simulink model "FLhighFidelityTiltingQuadrotor"  (R2022b)
settings: Solver=ode4  StartTime=0.0  StopTime=15  FixedStep=T_s  RelTol=1e-3
InitFcn:
  | run initFLhighFidelityTiltingQuadrotor
values from neighbouring files (symbols this model uses):
  kh1 = 1    [initFLhighFidelityTiltingQuadrotor.m]
  kh2 = 2    [initFLhighFidelityTiltingQuadrotor.m]
  Ts_st = settings.Ts_st    [initNMPChighFidelityTiltingQuadrotor.m]
  w_bar2_min = (0.01*prop.w_max).^2    [initFLhighFidelityTiltingQuadrotor.m]
  w_bar2_rest = tiltq.w_bar_hover_planar.^2    [initFLhighFidelityTiltingQuadrotor.m]
  w_bar_0 = w_bar_0(1:tiltq.N)    [highFidelityTiltingQuadrotorData.m]
undefined symbols (not defined in the file or in its folder): body, FL, prop, rad, s, tiltq
libraries: robotcorelib x4, simulink_extras x4, slpidlib x2, aerolibconvert2 x1, matrix_library x1
settings Model: PauseTimes=2  Creator=chen  LastModifiedBy=beniamino
settings SolverCC: AlgebraicLoopSolver=TrustRegion
settings DataIOCC: ReturnWorkspaceOutputs=off
settings DebuggingCC: UnconnectedInputMsg=warning  UnconnectedOutputMsg=warning  UnconnectedLineMsg=warning  SFMachineParentedDataDiag=warning  ArithmeticOperatorsInVariantConditions=warning
settings ModelReferenceCC: EnableRefExpFcnMdlSchedulingChecks=on
settings SFSimCC: SimUseLocalCustomCode=off  CustomCodeUndefinedFunction=UseInterfaceOnly
settings RTWCC: RTWUseLocalCustomCode=off  CheckMdlBeforeBuild=Error

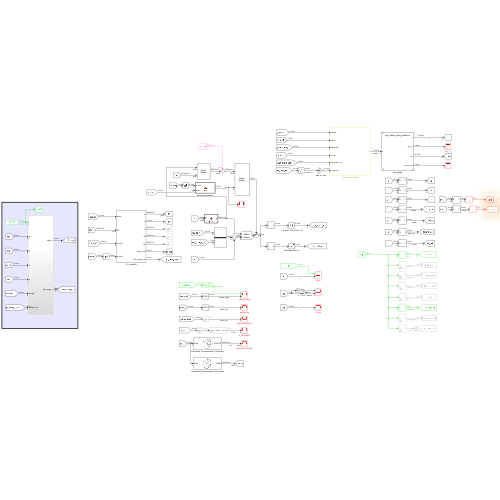
[thumbnail: Simulink's stored preview of the top-level diagram]
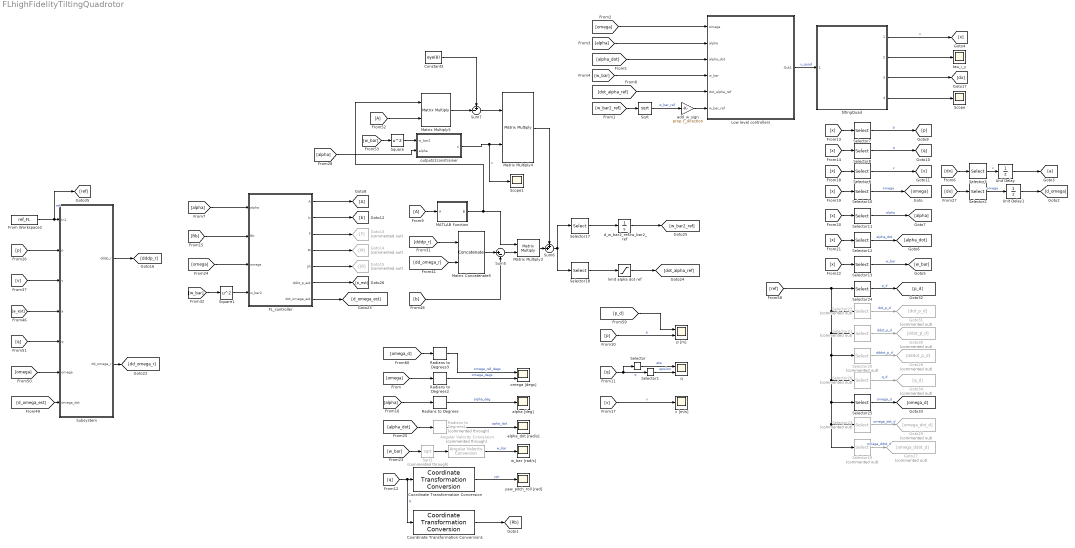
== system FLhighFidelityTiltingQuadrotor ==
  Angular Velocity Conversion : aerolibconvert2/Angular Velocity Conversion  Commented=through  IU=rad/s  OU=rpm
  Constant3 : Constant  Value=eye(8)
  Coordinate Transformation Conversion : robotcorelib/Coordinate Transformation Conversion  InputRepresentation=Quaternion  InputEulerSequence=ZYX  ShowTrVecInputPort=on  OutputRepresentation=Euler Angles  OutputEulerSequence=ZYX  ShowTrVecOutputPort=on  SimulateUsing=Code generation
  Coordinate Transformation Conversion1 : robotcorelib/Coordinate Transformation Conversion  InputRepresentation=Quaternion  InputEulerSequence=ZYX  ShowTrVecInputPort=on  OutputRepresentation=Rotation Matrix  OutputEulerSequence=ZYX  ShowTrVecOutputPort=on  SimulateUsing=Interpreted execution
  FL_controller : Subsystem
  From Workspace2 : FromWorkspace  VariableName=ref_FL  SampleTime=Ts_st
  From52 : From
  From9 : From
  Goto13 : Goto  Commented=on  GotoTag=F
  Goto14 : Goto  Commented=on  GotoTag=M
  Goto15 : Goto  Commented=on  GotoTag=JR
  Goto27 : Goto  Commented=on  GotoTag=omega_ddot_d
  Goto28 : Goto  Commented=on  GotoTag=dddot_p_d
  Goto29 : Goto  Commented=on  GotoTag=omega_dot_d
  Goto30 : Goto  Commented=on  GotoTag=ddot_p_d
  Goto31 : Goto  Commented=on  GotoTag=dot_p_d
  Goto34 : Goto  Commented=on  GotoTag=q_d
  Goto8 : Goto
  Low level controllers : Subsystem
  MATLAB Function : MATLAB Function  TreatAsAtomicUnit=on
  Matrix Concatenate5 : Concatenate  ConcatenateDimension=2
  Matrix Multiply3 : Product  Multiplication=Matrix(*)
  Matrix Multiply4 : Product  Multiplication=Matrix(*)
  Matrix Multiply5 : Product  Multiplication=Matrix(*)
  Radians to Degrees : simulink_extras/Transformations/Radians to Degrees
  Radians to Degrees1 : simulink_extras/Transformations/Radians to Degrees  Commented=through
  Radians to Degrees2 : simulink_extras/Transformations/Radians to Degrees
  Radians to Degrees3 : simulink_extras/Transformations/Radians to Degrees
  Scope : Scope
  Scope1 : Scope
  Selector : Selector  InputPortWidth=4  IndexOptions=Index vector (dialog)  Indices=1  OutputSizes=1
  Selector1 : Selector  InputPortWidth=4  IndexOptions=Index vector (dialog)  Indices=2:4  OutputSizes=1
  Selector10 : Selector  InputPortWidth=25  IndexOptions=Index vector (dialog)  Indices=11:13  OutputSizes=1
  Selector11 : Selector  InputPortWidth=25  IndexOptions=Index vector (dialog)  Indices=14:17  OutputSizes=1
  Selector12 : Selector  InputPortWidth=25  IndexOptions=Index vector (dialog)  Indices=18:21  OutputSizes=1
  Selector13 : Selector  InputPortWidth=25  IndexOptions=Index vector (dialog)  Indices=22:25  OutputSizes=1
  Selector17 : Selector  InputPortWidth=8  IndexOptions=Index vector (dialog)  Indices=1:4  OutputSizes=1
  Selector18 : Selector  InputPortWidth=8  IndexOptions=Index vector (dialog)  Indices=5:8  OutputSizes=1
  Selector19 : Selector  Commented=on  InputPortWidth=25  IndexOptions=Index vector (dialog)  Indices=23:25  OutputSizes=1
  Selector2 : Selector  InputPortWidth=25  IndexOptions=Index vector (dialog)  Indices=11:13  OutputSizes=1
  Selector20 : Selector  Commented=on  InputPortWidth=25  IndexOptions=Index vector (dialog)  Indices=20:22  OutputSizes=1
  Selector21 : Selector  Commented=on  InputPortWidth=25  IndexOptions=Index vector (dialog)  Indices=14:16  OutputSizes=1
  Selector22 : Selector  Commented=on  InputPortWidth=25  IndexOptions=Index vector (dialog)  Indices=8:10  OutputSizes=1
  Selector23 : Selector  Commented=on  InputPortWidth=25  IndexOptions=Index vector (dialog)  Indices=17:19  OutputSizes=1
  Selector24 : Selector  InputPortWidth=25  IndexOptions=Index vector (dialog)  Indices=1:3  OutputSizes=1
  Selector25 : Selector  InputPortWidth=25  IndexOptions=Index vector (dialog)  Indices=11:13  OutputSizes=1
  Selector26 : Selector  Commented=on  InputPortWidth=25  IndexOptions=Index vector (dialog)  Indices=4:7  OutputSizes=1
  Selector3 : Selector  InputPortWidth=25  IndexOptions=Index vector (dialog)  Indices=8:10  OutputSizes=1
  Selector7 : Selector  InputPortWidth=25  IndexOptions=Index vector (dialog)  Indices=1:3  OutputSizes=1
  Selector8 : Selector  InputPortWidth=25  IndexOptions=Index vector (dialog)  Indices=4:7  OutputSizes=1
  Selector9 : Selector  InputPortWidth=25  IndexOptions=Index vector (dialog)  Indices=8:10  OutputSizes=1
  Sqrt : Sqrt
  Sqrt1 : Sqrt  Commented=through
  Square : Math  Operator=square
  Square1 : Math  Operator=square
  Subsystem : Subsystem
  Sum5 : Sum  Inputs=|+-
  Sum6 : Sum  Inputs=++|
  Sum7 : Sum  Inputs=+-|
  Unit Delay : UnitDelay  SampleTime=-1  HasFrameUpgradeWarning=on
  Unit Delay1 : UnitDelay  SampleTime=-1  HasFrameUpgradeWarning=on
  add_w_sign : Gain  Gain=prop.c_direction
  alpha [deg] : Scope
  alpha_dot [rad/s] : Scope
  d_w_bar2_ref2w_bar2_ref : Integrator  InitialCondition=w_bar_0.^2  LimitOutput=on  UpperSaturationLimit=prop.w_max.^2  LowerSaturationLimit=prop.w_min.^2
  limit alpha dot ref : Saturate  UpperLimit=6  LowerLimit=-6
  omega [degs] : Scope  NumInputPorts=2
  outputs2constrainer : MATLAB Function  TreatAsAtomicUnit=on
  p [m] : Scope  NumInputPorts=2
  q : Scope  NumInputPorts=2
  tau_i_y : Scope
  tiltingQuad : Subsystem  ReferencedSubsystem=high_fidelity_tilting_quadrotor  p0=p_0  q0=q_0  v0=v_0  omega0=omega_0  alpha0=alpha_0  d_alpha_0=alpha_dot_0  bar_w0=w_bar_0  m_b=tiltq.m_b  beta=tiltq.beta  I_b=body.I  I_i=tiltq.I_i  c_direction=prop.c_direction  k_m=prop.k_m  k_t=prop.k_t  p_mot=tiltq.p_mot  min_alpha=tiltq.min_alpha  max_alpha=tiltq.max_alpha  min_d_alpha=tiltq.min_alpha_dot  max_d_alpha=tiltq.max_alpha_dot  min_bar_w=[prop.w_min prop.w_min -prop.w_max -prop.w_max]  max_bar_w=[prop.w_max prop.w_max -prop.w_min -prop.w_min]
  v [m/s] : Scope
  w_bar [rad/s] : Scope
  yaw_pitch_roll [rad] : Scope
  wires:
  tiltingQuad/3 -> [dx]
  tiltingQuad/1 -> [x]  "x"
  tiltingQuad/2 -> tau_i_y/1
  tiltingQuad/4 -> Scope/1
  [w_bar2_ref] -> Sqrt/1
  [omega] -> Low level controllers/1(omega)
  [alpha] -> Low level controllers/2(alpha)
  [alpha_dot] -> Low level controllers/3(alpha_dot)
  [w_bar] -> Low level controllers/4(w_bar)
  Sqrt/1 -> add_w_sign/1  "w_bar_ref"
  Low level controllers/1(Out1) -> tiltingQuad/1  "u_quad"
  [dot_alpha_ref] -> Low level controllers/5(dot_alpha_ref)
  Sum5/1 -> Matrix Multiply3/2
  Selector17/1 -> d_w_bar2_ref2w_bar2_ref/1
  MATLAB Function/1(B) -> Matrix Multiply5/1, Matrix Multiply3/1
  From Workspace2/1 -> [ref], Subsystem/1(In1)  "ref"
  [b] -> Sum5/2
  [p_d] -> p [m]/1
  [alpha] -> FL_controller/1(alpha)
  [q] -> Coordinate Transformation Conversion1/1, Coordinate Transformation Conversion/1  "q"
  Sqrt1/1 -> Angular Velocity Conversion/1
  [a_est] -> Subsystem/4(a)
  [p] -> Subsystem/2(p)
  Selector1/1 -> q/2  "epsilon"
  From9/1 -> MATLAB Function/1(A)
  Radians to Degrees2/1 -> omega [degs]/2  "omega_degs"
  Selector13/1 -> [w_bar]  "w_bar"
  Selector11/1 -> [alpha]  "alpha"
  [alpha] -> Radians to Degrees/1
  Subsystem/2(dd_omega_r) -> [dd_omega_r]
  Sum6/1 -> Selector18/1, Selector17/1
  [q] -> Selector1/1, Selector/1  "q"
  [w_bar] -> Square1/1
  [omega] -> Radians to Degrees2/1
  FL_controller/2(b) -> [b]
  [x] -> Selector10/1
  [x] -> Selector8/1
  Radians to Degrees/1 -> alpha [deg]/1  "alpha_deg"
  [v] -> Subsystem/3(v)
  Radians to Degrees1/1 -> alpha_dot [rad/s]/1  "apha_dot"
  Selector9/1 -> [v]  "v"
  [dd_omega_r] -> Matrix Concatenate5/2
  [x] -> Selector9/1
  Coordinate Transformation Conversion1/1 -> [Rb]
  FL_controller/1(A) -> Goto8/1
  FL_controller/3(F) -> Goto13/1
  Selector/1 -> q/1  "eta"
  Selector10/1 -> [omega]  "omega"
  Matrix Multiply5/1 -> Sum7/2
  Selector12/1 -> [alpha_dot]  "alpha_dot"
  Selector7/1 -> [p]  "p"
  [p] -> p [m]/2  "p"
  Matrix Concatenate5/1 -> Sum5/1
  [w_bar] -> Square/1
  Angular Velocity Conversion/1 -> w_bar [rad/s]/1  "w_bar"
  [x] -> Selector11/1
  Subsystem/1(dddp_r) -> [dddp_r]
  [x] -> Selector7/1
  Coordinate Transformation Conversion/1 -> yaw_pitch_roll [rad]/1  "ypr"
  Selector20/1 -> Goto28/1  "dddot_p_d"
  [Rb] -> FL_controller/2(Rb)
  From52/1 -> Matrix Multiply5/2
  [omega] -> FL_controller/3(omega)
  [x] -> Selector13/1
  Constant3/1 -> Sum7/1
  [alpha_dot] -> Radians to Degrees1/1
  Selector18/1 -> limit alpha dot ref/1
  FL_controller/5(JR) -> Goto15/1
  [d_omega_est] -> Subsystem/7(omega_dot)
  Selector24/1 -> [p_d]  "p_d"
  FL_controller/7(dot_omega_est) -> [d_omega_est]
  [x] -> Selector12/1
  [w_bar] -> Sqrt1/1
  [dddp_r] -> Matrix Concatenate5/1
  Matrix Multiply3/1 -> Sum6/2
  Sum7/1 -> Matrix Multiply4/1
  [v] -> v [m/s]/1  "v"
  Matrix Multiply4/1 -> Sum6/1
  [omega] -> Subsystem/6(omega)
  Selector26/1 -> Goto34/1  "q_d"
  outputs2constrainer/1(z) -> Scope1/1, Matrix Multiply4/2  "z"
  [ref] -> Selector21/1, Selector26/1, Selector25/1, Selector19/1, Selector23/1, Selector20/1, Selector22/1, Selector24/1
  Selector23/1 -> Goto29/1  "omega_dot_d"
  Selector8/1 -> [q]  "q"
  Selector21/1 -> Goto30/1  "ddot_p_d"
  FL_controller/6(ddot_p_est) -> [a_est]
  [q] -> Subsystem/5(q)
  FL_controller/4(M) -> Goto14/1
  Selector19/1 -> Goto27/1  "omega_ddot_d"
  [omega_d] -> Radians to Degrees3/1
  d_w_bar2_ref2w_bar2_ref/1 -> [w_bar2_ref]
  Selector25/1 -> [omega_d]  "omega_d"
  Selector22/1 -> Goto31/1  "dot_p_d"
  Radians to Degrees3/1 -> omega [degs]/1  "omega_ref_degs"
  add_w_sign/1 -> Low level controllers/6(w_bar_ref)
  Square/1 -> outputs2constrainer/1(w_bar2)
  Square1/1 -> FL_controller/4(w_bar2)
  limit alpha dot ref/1 -> [dot_alpha_ref]
  Selector2/1 -> Unit Delay1/1  "omega"
  [dx] -> Selector3/1
  Selector3/1 -> Unit Delay/1  "v"
  [dx] -> Selector2/1
  Unit Delay/1 -> [a]
  Unit Delay1/1 -> [d_omega]
  [alpha] -> outputs2constrainer/2(alpha)

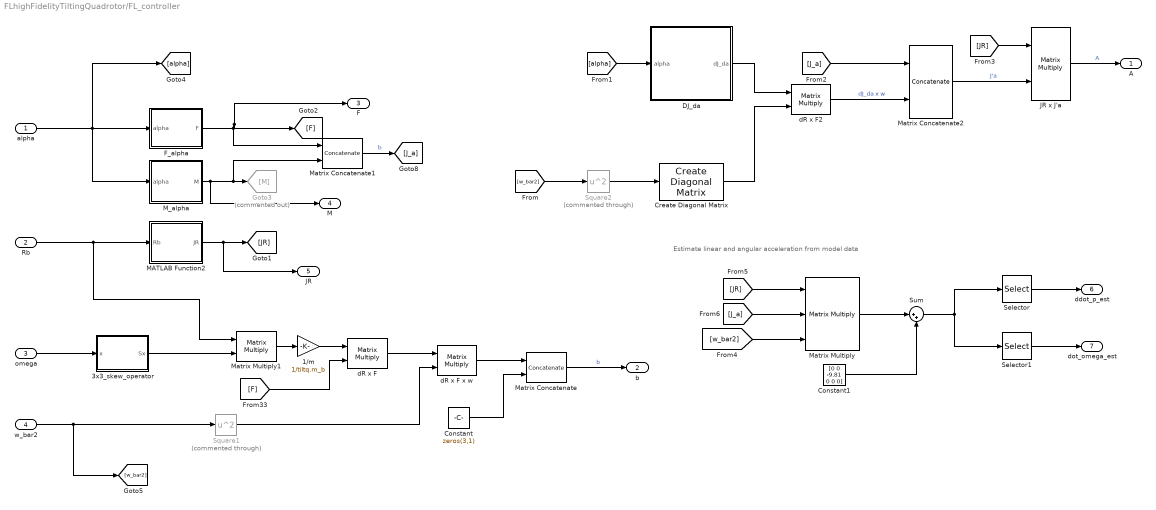
== system FLhighFidelityTiltingQuadrotor/FL_controller ==
  note: Estimate linear and angular acceleration from model data
  alpha : Inport
  Rb : Inport  Port=2
  omega : Inport  Port=3
  w_bar2 : Inport  Port=4
  1/m : Gain  Gain=1/tiltq.m_b
  3x3_skew_operator : MATLAB Function  TreatAsAtomicUnit=on
  Constant : Constant  Value=zeros(3,1)
  Constant1 : Constant  Value=[0 0 -9.81 0 0 0]
  Create Diagonal Matrix : matrix_library/Create Diagonal Matrix
      settings: LibrarySourceBlock=|
      | simulink/Matrix
      | Operations/Create Diagonal
      | Matrix
  DJ_da : MATLAB Function  TreatAsAtomicUnit=on  mask{c_t=prop.k_t, c_tau=prop.k_m, p_mot=tiltq.p_mot, beta=tiltq.beta, c_d=-prop.c_direction}
      mask prompts: c_t "thrust const"; c_tau "drag const"; p_mot "motor positions"; c_d "spinning directions"
  F_alpha : MATLAB Function  TreatAsAtomicUnit=on  mask{beta=tiltq.beta, c_t=prop.k_t}
      mask prompts: c_t "thrust_coeff"
  Goto3 : Goto  Commented=on  GotoTag=M
  JR x J'a : Product  Multiplication=Matrix(*)
  MATLAB Function2 : MATLAB Function  TreatAsAtomicUnit=on  mask{m=tiltq.m_b, Ib=body.I}
      mask prompts: m "mass"; Ib "Body inertia"
  M_alpha : MATLAB Function  TreatAsAtomicUnit=on  mask{beta=tiltq.beta, theta=tiltq.theta, c_t=prop.k_t, c_tau=prop.k_m, c_direction=-prop.c_direction, p_mot=tiltq.p_mot}
      mask prompts: c_t "thrust coeff"; c_tau "drag coeff"; c_direction "spinning dir"; p_mot "motor pos"
  Matrix Concatenate : Concatenate  Mode=Multidimensional array
  Matrix Concatenate1 : Concatenate  Mode=Multidimensional array
  Matrix Concatenate2 : Concatenate  Mode=Multidimensional array  ConcatenateDimension=2
  Matrix Multiply : Product  Inputs=3  Multiplication=Matrix(*)
  Matrix Multiply1 : Product  Multiplication=Matrix(*)
  Selector : Selector  InputPortWidth=6  IndexOptions=Index vector (dialog)  Indices=1:3  OutputSizes=1
  Selector1 : Selector  InputPortWidth=6  IndexOptions=Index vector (dialog)  Indices=4:6  OutputSizes=1
  Square1 : Math  Commented=through  Operator=square
  Square2 : Math  Commented=through  Operator=square
  Sum : Sum  Inputs=|++
  dR x F : Product  Multiplication=Matrix(*)
  dR x F x w : Product  Multiplication=Matrix(*)
  dR x F2 : Product  Multiplication=Matrix(*)
  A : Outport  PortDimensions=[6 8]
  b : Outport  Port=2  PortDimensions=6
  F : Outport  Port=3
  M : Outport  Port=4
  JR : Outport  Port=5
  ddot_p_est : Outport  Port=6
  dot_omega_est : Outport  Port=7
  wires:
  dR x F/1 -> dR x F x w/1
  dR x F x w/1 -> Matrix Concatenate/1
  Constant/1 -> Matrix Concatenate/2
  1/m/1 -> dR x F/1
  Rb/1 -> Matrix Multiply1/1, MATLAB Function2/1(Rb)
  M_alpha/1(M) -> M/1, Matrix Concatenate1/2, Goto3/1
  3x3_skew_operator/1(Sx) -> Matrix Multiply1/2
  alpha/1 -> [alpha], M_alpha/1(alpha), F_alpha/1(alpha)
  omega/1 -> 3x3_skew_operator/1(x)
  Square1/1 -> dR x F x w/2
  Matrix Concatenate1/1 -> [J_a]  "b"
  [F] -> dR x F/2
  w_bar2/1 -> [w_bar2], Square1/1
  MATLAB Function2/1(JR) -> JR/1, [JR]
  F_alpha/1(F) -> F/1, [F], Matrix Concatenate1/1
  Matrix Multiply1/1 -> 1/m/1
  Matrix Concatenate/1 -> b/1  "b"
  [J_a] -> Matrix Concatenate2/1
  Matrix Concatenate2/1 -> JR x J'a/2  "J'a"
  [JR] -> JR x J'a/1
  JR x J'a/1 -> A/1  "A"
  [w_bar2] -> Square2/1
  DJ_da/1(dJ_da) -> dR x F2/1
  [alpha] -> DJ_da/1(alpha)
  dR x F2/1 -> Matrix Concatenate2/2  "dJ_da x w"
  Square2/1 -> Create Diagonal Matrix/1
  Create Diagonal Matrix/1 -> dR x F2/2
  [w_bar2] -> Matrix Multiply/3
  [JR] -> Matrix Multiply/1
  [J_a] -> Matrix Multiply/2
  Matrix Multiply/1 -> Sum/1
  Selector/1 -> ddot_p_est/1
  Selector1/1 -> dot_omega_est/1
  Sum/1 -> Selector/1, Selector1/1
  Constant1/1 -> Sum/2

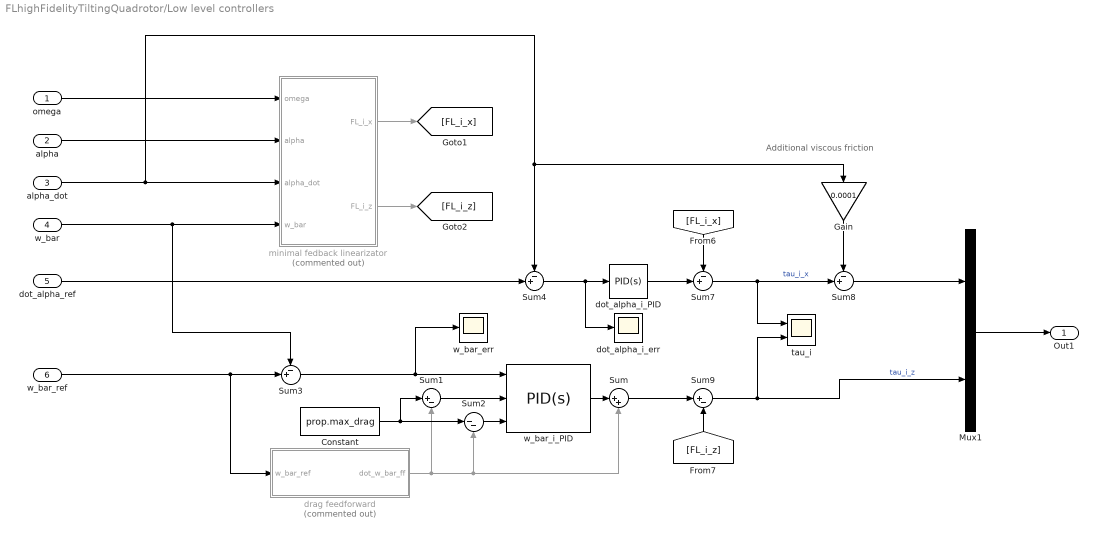
== system FLhighFidelityTiltingQuadrotor/Low level controllers ==
  note: Additional viscous friction
  omega : Inport
  alpha : Inport  Port=2
  alpha_dot : Inport  Port=3
  w_bar : Inport  Port=4
  dot_alpha_ref : Inport  Port=5
  w_bar_ref : Inport  Port=6
  Constant : Constant  Value=prop.max_drag
  Gain : Gain  Gain=0.0001
  Mux1 : Mux  Inputs=2
  Sum : Sum  Inputs=|++
  Sum1 : Sum  Inputs=|+-
  Sum2 : Sum  Inputs=|--
  Sum{3..4,7..8} (4 alike) : Sum  Inputs=-+|
  Sum9 : Sum  Inputs=|+-
  dot_alpha_i_PID : slpidlib/PID Controller  Controller=PID  Form=Parallel  TimeDomain=Continuous-time  UseExternalTs=off  SampleTime=-1  IntegratorMethod=Forward Euler  FilterMethod=Forward Euler  ControllerParametersSource=internal  P=0.01  I=0.1  UseKiTs=off  D=0.00001  N=100  UseFilter=on  TunerSelectOption=Transfer Function Based (PID Tuner App)  InitialConditionSource=internal  InitialConditionForIntegrator=0  InitialConditionForFilter=0  DifferentiatorICPrevScaledInput=0  ExternalReset=none  TrackingMode=off  Kt=1  LimitOutput=off  SatLimitsSource=internal  UpperSaturationLimit=6  LowerSaturationLimit=-6  LinearizeAsGain=on  AntiWindupMode=back-calculation  Kb=1  LimitIntegrator=off  UpperIntegratorSaturationLimit=inf  LowerIntegratorSaturationLimit=-inf  POutMin=[]  POutMax=[]  IOutMin=[]  IOutMax=[]  DOutMin=[]  DOutMax=[]  NOutMin=[]  NOutMax=[]  SumOutMin=[]  SumOutMax=[]  SaturationOutMin=[]  SaturationOutMax=[]  PParamMin=[]  PParamMax=[]  IParamMin=[]  IParamMax=[]  DParamMin=[]  DParamMax=[]  NParamMin=[]  NParamMax=[]  KbParamMin=[]  KbParamMax=[]  KtParamMin=[]  KtParamMax=[]  KbOutMin=[]  KbOutMax=[]  KtOutMin=[]  KtOutMax=[]  IntegratorOutMin=[]  IntegratorOutMax=[]  FilterOutMin=[]  FilterOutMax=[]  SumI1OutMin=[]  SumI1OutMax=[]  SumI2OutMin=[]  SumI2OutMax=[]  SumI3OutMin=[]  SumI3OutMax=[]  SumI4OutMin=[]  SumI4OutMax=[]  SumDOutMin=[]  SumDOutMax=[]  DifferentiatorOutMin=[]  DifferentiatorOutMax=[]  FilterDiffOutCoefMin=[]  FilterDiffOutCoefMax=[]  ReciprocalOutMin=[]  ReciprocalOutMax=[]  SumDenOutMin=[]  SumDenOutMax=[]  SumNumOutMin=[]  SumNumOutMax=[]  DivideOutMin=[]  DivideOutMax=[]  UdiffTsProdOutMin=[]  UdiffTsProdOutMax=[]  NTsProdOutMin=[]  NTsProdOutMax=[]  UintegralTsProdOutMin=[]  UintegralTsProdOutMax=[]  UngainTsProdOutMin=[]  UngainTsProdOutMax=[]  ClampingZeroOutDataTypeStr=Inherit: Inherit via back propagation  ClampingZeroOutMin=[]  ClampingZeroOutMax=[]  FilterDenConstantOutDataTypeStr=Inherit: Inherit via back propagation  FilterDenConstantOutMin=[]  FilterDenConstantOutMax=[]  PCopyOutDataTypeStr=Inherit: Inherit via back propagation  PCopyOutMin=[]  PCopyOutMax=[]  NCopyOutDataTypeStr=Inherit: Inherit via back propagation  NCopyOutMin=[]  NCopyOutMax=[]  IntegratorContinuousStateAttributes=''  IntegratorStateMustResolveToSignalObject=off  IntegratorRTWStateStorageClass=Auto  FilterContinuousStateAttributes=''  FilterStateMustResolveToSignalObject=off  FilterRTWStateStorageClass=Auto  ParallelPVariant=InternalParameters  IdealPVariant=Disabled  IVariant=InternalParameters  DVariant=InternalParameters  IntegratorVariant=Continuous  SatVariant=Disabled  AWVariant=Passthrough  PCopyVariant=Disabled  TRVariant=Disabled  FdbkBlocksVariant=Forward  IdealPFdbkVariant=Disabled  SatFdbkVariant=Disabled  DerivativeFilterVariant=ContFilter  NVariant=InternalParameters  NCopyVariant=Disabled  FilterICVariant=InternalICsFilter  IntegratorICVariant=InternalICs  ExternalResetVariant=Disabled  TRSumVariant=Passthrough  SumFdbkVariant=Disabled  SumVariant=Sum_PID  TsampFilterVariant=InternalTs  TsampNgainVariant=Passthrough  TsampIntegralVariant=Passthrough  ExternalSaturationOutDataTypeStr=Inherit: Same as second input
  dot_alpha_i_err : Scope
  drag feedforward : MATLAB Function  Commented=on  TreatAsAtomicUnit=on  mask{k_m=prop.k_m}
      mask prompts: k_m "motor drag constant"
  minimal fedback linearizator : MATLAB Function  Commented=on  TreatAsAtomicUnit=on  mask{N=tiltq.N, I_i=tiltq.I_i, beta=tiltq.beta}
      mask prompts: N "number of propellers"; I_i "propeller + rotor inertia matrix"; beta "propeller tilting planes angles"
  tau_i : Scope  NumInputPorts=2
  w_bar_err : Scope
  w_bar_i_PID : slpidlib/PID Controller  Controller=PID  Form=Parallel  TimeDomain=Continuous-time  UseExternalTs=off  SampleTime=-1  IntegratorMethod=Forward Euler  FilterMethod=Forward Euler  ControllerParametersSource=internal  P=0.01  I=0.1  UseKiTs=on  D=0.00001  N=100  UseFilter=on  TunerSelectOption=Transfer Function Based (PID Tuner App)  InitialConditionSource=internal  InitialConditionForIntegrator=0  InitialConditionForFilter=0  DifferentiatorICPrevScaledInput=0  ExternalReset=none  TrackingMode=off  Kt=1  LimitOutput=on  SatLimitsSource=external  UpperSaturationLimit=inf  LowerSaturationLimit=-inf  LinearizeAsGain=on  AntiWindupMode=back-calculation  Kb=10  LimitIntegrator=off  UpperIntegratorSaturationLimit=inf  LowerIntegratorSaturationLimit=-inf  POutMin=[]  POutMax=[]  IOutMin=[]  IOutMax=[]  DOutMin=[]  DOutMax=[]  NOutMin=[]  NOutMax=[]  SumOutMin=[]  SumOutMax=[]  SaturationOutMin=[]  SaturationOutMax=[]  PParamMin=[]  PParamMax=[]  IParamMin=[]  IParamMax=[]  DParamMin=[]  DParamMax=[]  NParamMin=[]  NParamMax=[]  KbParamMin=[]  KbParamMax=[]  KtParamMin=[]  KtParamMax=[]  KbOutMin=[]  KbOutMax=[]  KtOutMin=[]  KtOutMax=[]  IntegratorOutMin=[]  IntegratorOutMax=[]  FilterOutMin=[]  FilterOutMax=[]  SumI1OutMin=[]  SumI1OutMax=[]  SumI2OutMin=[]  SumI2OutMax=[]  SumI3OutMin=[]  SumI3OutMax=[]  SumI4OutMin=[]  SumI4OutMax=[]  SumDOutMin=[]  SumDOutMax=[]  DifferentiatorOutMin=[]  DifferentiatorOutMax=[]  FilterDiffOutCoefMin=[]  FilterDiffOutCoefMax=[]  ReciprocalOutMin=[]  ReciprocalOutMax=[]  SumDenOutMin=[]  SumDenOutMax=[]  SumNumOutMin=[]  SumNumOutMax=[]  DivideOutMin=[]  DivideOutMax=[]  UdiffTsProdOutMin=[]  UdiffTsProdOutMax=[]  NTsProdOutMin=[]  NTsProdOutMax=[]  UintegralTsProdOutMin=[]  UintegralTsProdOutMax=[]  UngainTsProdOutMin=[]  UngainTsProdOutMax=[]  ClampingZeroOutDataTypeStr=Inherit: Inherit via back propagation  ClampingZeroOutMin=[]  ClampingZeroOutMax=[]  FilterDenConstantOutDataTypeStr=Inherit: Inherit via back propagation  FilterDenConstantOutMin=[]  FilterDenConstantOutMax=[]  PCopyOutDataTypeStr=Inherit: Inherit via back propagation  PCopyOutMin=[]  PCopyOutMax=[]  NCopyOutDataTypeStr=Inherit: Inherit via back propagation  NCopyOutMin=[]  NCopyOutMax=[]  IntegratorContinuousStateAttributes=''  IntegratorStateMustResolveToSignalObject=off  IntegratorRTWStateStorageClass=Auto  FilterContinuousStateAttributes=''  FilterStateMustResolveToSignalObject=off  FilterRTWStateStorageClass=Auto  ParallelPVariant=InternalParameters  IdealPVariant=Disabled  IVariant=InternalParameters  DVariant=InternalParameters  IntegratorVariant=Continuous  SatVariant=External  AWVariant=BackCalculation  PCopyVariant=Disabled  TRVariant=Disabled  FdbkBlocksVariant=Forward  IdealPFdbkVariant=Disabled  SatFdbkVariant=Disabled  DerivativeFilterVariant=ContFilter  NVariant=InternalParameters  NCopyVariant=Disabled  FilterICVariant=InternalICsFilter  IntegratorICVariant=InternalICs  ExternalResetVariant=Disabled  TRSumVariant=Passthrough  SumFdbkVariant=Disabled  SumVariant=Sum_PID  TsampFilterVariant=InternalTs  TsampNgainVariant=Passthrough  TsampIntegralVariant=Passthrough  ExternalSaturationOutDataTypeStr=Inherit: Same as second input
  Out1 : Outport
  wires:
  Sum2/1 -> w_bar_i_PID/3
  w_bar_i_PID/1 -> Sum/1
  minimal fedback linearizator/1(FL_i_x) -> [FL_i_x]
  Sum8/1 -> Mux1/1
  dot_alpha_i_PID/1 -> Sum7/2
  alpha_dot/1 -> Gain/1, Sum4/1, minimal fedback linearizator/3(alpha_dot)
  Sum4/1 -> dot_alpha_i_err/1, dot_alpha_i_PID/1
  [FL_i_z] -> Sum9/2
  minimal fedback linearizator/2(FL_i_z) -> [FL_i_z]
  alpha/1 -> minimal fedback linearizator/2(alpha)
  Sum9/1 -> tau_i/2, Mux1/2  "tau_i_z"
  omega/1 -> minimal fedback linearizator/1(omega)
  Sum/1 -> Sum9/1
  Sum1/1 -> w_bar_i_PID/2
  [FL_i_x] -> Sum7/1
  Mux1/1 -> Out1/1
  Sum3/1 -> w_bar_err/1, w_bar_i_PID/1
  w_bar/1 -> Sum3/1, minimal fedback linearizator/4(w_bar)
  dot_alpha_ref/1 -> Sum4/2
  Sum7/1 -> tau_i/1, Sum8/2  "tau_i_x"
  Gain/1 -> Sum8/1
  w_bar_ref/1 -> Sum3/2, drag feedforward/1(w_bar_ref)
  drag feedforward/1(dot_w_bar_ff) -> Sum/2, Sum2/2, Sum1/2
  Constant/1 -> Sum2/1, Sum1/1

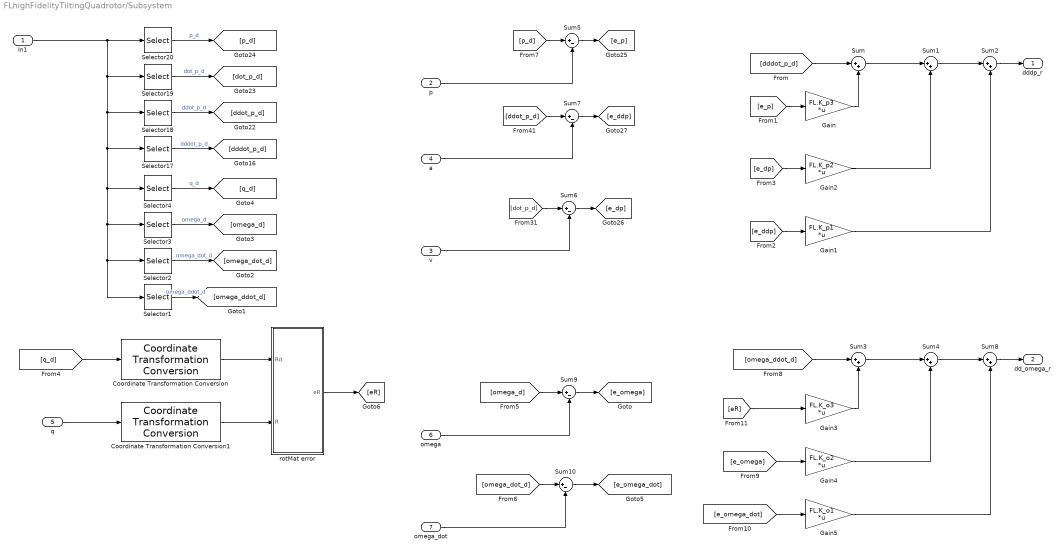
== system FLhighFidelityTiltingQuadrotor/Subsystem ==
  In1 : Inport
  p : Inport  Port=2
  v : Inport  Port=3
  a : Inport  Port=4
  q : Inport  Port=5
  omega : Inport  Port=6
  omega_dot : Inport  Port=7
  Coordinate Transformation Conversion : robotcorelib/Coordinate Transformation Conversion  InputRepresentation=Quaternion  InputEulerSequence=ZYX  ShowTrVecInputPort=on  OutputRepresentation=Rotation Matrix  OutputEulerSequence=ZYX  ShowTrVecOutputPort=on  SimulateUsing=Interpreted execution
  Coordinate Transformation Conversion1 : robotcorelib/Coordinate Transformation Conversion  InputRepresentation=Quaternion  InputEulerSequence=ZYX  ShowTrVecInputPort=on  OutputRepresentation=Rotation Matrix  OutputEulerSequence=ZYX  ShowTrVecOutputPort=on  SimulateUsing=Interpreted execution
  Gain : Gain  Gain=FL.K_p3  Multiplication=Matrix(K*u) (u vector)
  Gain1 : Gain  Gain=FL.K_p1  Multiplication=Matrix(K*u) (u vector)
  Gain2 : Gain  Gain=FL.K_p2  Multiplication=Matrix(K*u) (u vector)
  Gain3 : Gain  Gain=FL.K_o3  Multiplication=Matrix(K*u) (u vector)
  Gain4 : Gain  Gain=FL.K_o2  Multiplication=Matrix(K*u) (u vector)
  Gain5 : Gain  Gain=FL.K_o1  Multiplication=Matrix(K*u) (u vector)
  Selector1 : Selector  InputPortWidth=25  IndexOptions=Index vector (dialog)  Indices=23:25  OutputSizes=1
  Selector17 : Selector  InputPortWidth=25  IndexOptions=Index vector (dialog)  Indices=20:22  OutputSizes=1
  Selector18 : Selector  InputPortWidth=25  IndexOptions=Index vector (dialog)  Indices=14:16  OutputSizes=1
  Selector19 : Selector  InputPortWidth=25  IndexOptions=Index vector (dialog)  Indices=8:10  OutputSizes=1
  Selector2 : Selector  InputPortWidth=25  IndexOptions=Index vector (dialog)  Indices=17:19  OutputSizes=1
  Selector20 : Selector  InputPortWidth=25  IndexOptions=Index vector (dialog)  Indices=1:3  OutputSizes=1
  Selector3 : Selector  InputPortWidth=25  IndexOptions=Index vector (dialog)  Indices=11:13  OutputSizes=1
  Selector4 : Selector  InputPortWidth=25  IndexOptions=Index vector (dialog)  Indices=4:7  OutputSizes=1
  Sum{,1..4,8} (6 alike) : Sum  Inputs=|++
  Sum{5..7,9..10} (5 alike) : Sum  Inputs=|+-
  rotMat error : MATLAB Function  TreatAsAtomicUnit=on
  dddp_r : Outport
  dd_omega_r : Outport  Port=2
  wires:
  Selector19/1 -> [dot_p_d]  "dot_p_d"
  a/1 -> Sum7/2
  [p_d] -> Sum5/1
  p/1 -> Sum5/2
  [ddot_p_d] -> Sum7/1
  Selector18/1 -> [ddot_p_d]  "ddot_p_d"
  Sum6/1 -> [e_dp]
  [dot_p_d] -> Sum6/1
  v/1 -> Sum6/2
  Sum7/1 -> [e_ddp]
  Sum5/1 -> [e_p]
  Selector17/1 -> [dddot_p_d]  "dddot_p_d"
  Selector20/1 -> [p_d]  "p_d"
  [dddot_p_d] -> Sum/1
  [e_p] -> Gain/1
  Gain/1 -> Sum/2
  Sum/1 -> Sum1/1
  [e_ddp] -> Gain1/1
  Gain1/1 -> Sum2/2
  [e_dp] -> Gain2/1
  Sum1/1 -> Sum2/1
  Gain2/1 -> Sum1/2
  Sum2/1 -> dddp_r/1
  Sum8/1 -> dd_omega_r/1
  Gain3/1 -> Sum3/2
  Gain5/1 -> Sum8/2
  Sum3/1 -> Sum4/1
  Gain4/1 -> Sum4/2
  Sum4/1 -> Sum8/1
  [omega_ddot_d] -> Sum3/1
  Selector4/1 -> [q_d]  "q_d"
  Selector1/1 -> [omega_ddot_d]  "omega_ddot_d"
  Selector2/1 -> [omega_dot_d]  "omega_dot_d"
  In1/1 -> Selector18/1, Selector4/1, Selector3/1, Selector1/1, Selector2/1, Selector17/1, Selector19/1, Selector20/1
  Selector3/1 -> [omega_d]  "omega_d"
  [omega_d] -> Sum9/1
  omega/1 -> Sum9/2
  [omega_dot_d] -> Sum10/1
  omega_dot/1 -> Sum10/2
  Sum9/1 -> [e_omega]
  Sum10/1 -> [e_omega_dot]
  [e_omega] -> Gain4/1
  [e_omega_dot] -> Gain5/1
  [q_d] -> Coordinate Transformation Conversion/1
  q/1 -> Coordinate Transformation Conversion1/1
  Coordinate Transformation Conversion/1 -> rotMat error/1(Rd)
  Coordinate Transformation Conversion1/1 -> rotMat error/2(R)
  rotMat error/1(eR) -> [eR]
  [eR] -> Gain3/1

== matlab function FLhighFidelityTiltingQuadrotor/outputs2constrainer ==
  data: w_bar2 input size=4; z output size=8; w_bar2_min parameter; w_bar2_rest parameter; kh1 parameter; kh2 parameter; alpha input
function z = fcn(w_bar2, w_bar2_min, w_bar2_rest, kh1, kh2, alpha)


gamma1 = pi/(2*(w_bar2_rest-w_bar2_min));
gamma2 = -gamma1*w_bar2_rest;


z=zeros(8,1);

for k=1:4
    if(w_bar2(k)<=w_bar2_rest)
        w2_tmp = gamma1*w_bar2(k)+gamma2;
        z(k) = -kh1 .* sec(w2_tmp).^2*tan(w2_tmp) .* gamma1;
    else
        w2_tmp = w_bar2(k)-w_bar2_rest;
        z(k) = -kh2 .* 2.*(w2_tmp);
    end
end

%z(5:8) = -1e10.*alpha.^7;

== matlab function FLhighFidelityTiltingQuadrotor/Low level controllers/drag feedforward ==
  data: w_bar_ref input; dot_w_bar_ff output; k_m parameter
function dot_w_bar_ff = fcn(w_bar_ref, k_m)

dot_w_bar_ff = k_m .* w_bar_ref .* abs(w_bar_ref);

== matlab function FLhighFidelityTiltingQuadrotor/MATLAB Function ==
  data: A input; B output
function B = pinv(A)

B = pinv(A);

== matlab function FLhighFidelityTiltingQuadrotor/Low level controllers/minimal fedback linearizator ==
  data: omega input; alpha input; FL_i_x output; beta parameter; N parameter; alpha_dot input; w_bar input; FL_i_z output; I_i parameter
function [FL_i_x, FL_i_z]= fcn(omega, alpha, beta, N, alpha_dot, w_bar, I_i)

FL_i_x = zeros(4,1);
FL_i_z = zeros(4,1);

for i=1:N
    B_R_i = axang2rotm([0 0 1 beta(i)])*axang2rotm([1 0 0 alpha(i)]);
    omega_i = B_R_i.' * omega + [alpha_dot(i); 0; w_bar(i)];
    coriol_i = cross(omega_i, I_i*omega_i);
    FF_i = coriol_i;
    FL_i_x(i) = -FF_i(1);
    FL_i_z(i) = -FF_i(3);
end

== matlab function FLhighFidelityTiltingQuadrotor/FL_controller/F_alpha ==
  data: alpha input; F output; beta parameter; c_t parameter
function F = F(alpha, beta, c_t)

F_temp= [...
    (sin(beta).*sin(alpha)).';...
    (-cos(beta).*sin(alpha)).';...
    (cos(alpha)).'];

F = c_t .* F_temp;

== matlab function FLhighFidelityTiltingQuadrotor/FL_controller/M_alpha ==
  data: alpha input; M output; beta parameter; theta parameter; c_t parameter; c_tau parameter; c_direction parameter; p_mot parameter
function M = M(alpha, beta, theta, c_t, c_tau, c_direction, p_mot)

delta = theta - beta;
l = vecnorm(p_mot,2,2);
F_temp= [...
    (sin(beta).*sin(alpha)).';...
    (-cos(beta).*sin(alpha)).';...
    (cos(alpha)).'];
M_drag = c_tau .* F_temp * diag(c_direction);
M_thrust = c_t .* [...
    (sin(theta).*cos(alpha)).';...
    (-cos(theta).*cos(alpha)).';...
    (-cos(delta).*sin(alpha)).']...
    *diag(l);
M = M_drag + M_thrust;

== matlab function FLhighFidelityTiltingQuadrotor/FL_controller/MATLAB Function2 ==
  data: Rb input; JR output; m parameter; Ib parameter
function JR = JR(Rb, m, Ib)

JR=[1/m.*Rb, zeros(3,3);
    zeros(3,3), inv(Ib)];

== matlab function FLhighFidelityTiltingQuadrotor/FL_controller/3x3_skew_operator ==
  data: x input; Sx output
function Sx = fcn(x)

Sx=[0 -x(3) x(2) ; x(3) 0 -x(1) ; -x(2) x(1) 0 ];

== matlab function FLhighFidelityTiltingQuadrotor/FL_controller/DJ_da ==
  data: alpha input; dJ_da output; beta parameter; c_t parameter; c_tau parameter; p_mot parameter; c_d parameter
function dJ_da = fcn(alpha, beta, c_t, c_tau, p_mot, c_d)

l = vecnorm(p_mot,2,2);

dF_da = c_t.*[(sin(beta).*cos(alpha)).';...
              (-cos(beta).*cos(alpha)).';...
              (-sin(alpha)).'];

dMd_da = c_tau.*[(sin(beta).*cos(alpha)).';...
                 (-cos(beta).*cos(alpha)).';...
                 (-sin(alpha)).']*diag(c_d);

dMt_da = c_t.*[(-sin(beta).*sin(alpha)).';...
               (cos(beta).*sin(alpha)).';...
               (-cos(alpha)).']*diag(l);

dJ_da = [dF_da;
         dMd_da + dMt_da];

== matlab function FLhighFidelityTiltingQuadrotor/Subsystem/rotMat error ==
  data: Rd input; eR output size=3; R input
function eR = fcn(Rd, R)

Re = 0.5*(R.'*Rd-Rd.'*R);

eR = zeros(3,1);
eR(1) = Re(3,2);
eR(2) = Re(1,3);
eR(3) = Re(2,1);
